simulink model "BDotv1"  (R2023b)
settings: Solver=FixedStepAuto  StartTime=0.0  StopTime=6000  FixedStep=1  RelTol=1e-3
undefined symbols (not defined in the file or in its folder): EIGEN, GL04C, IAU
libraries: aerolibtransform2 x3, aerolibutil x3, sharedutil x1, vrlib x1
settings Model: Creator=moonr  LastModifiedBy=moonr
settings HardwareCC: ProdBitPerLong=64  ProdLargestAtomicFloat=None  ProdHWDeviceType=AMD->Athlon 64

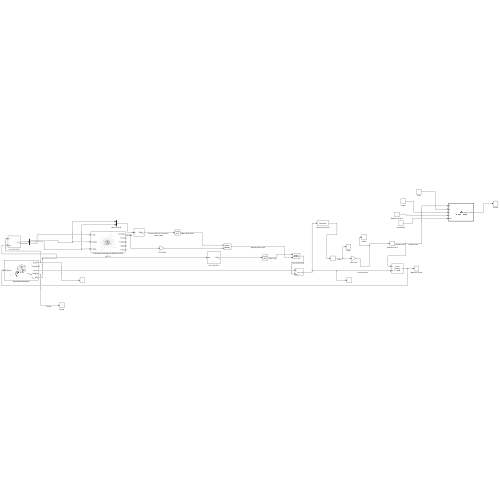
[thumbnail: Simulink's stored preview of the top-level diagram]
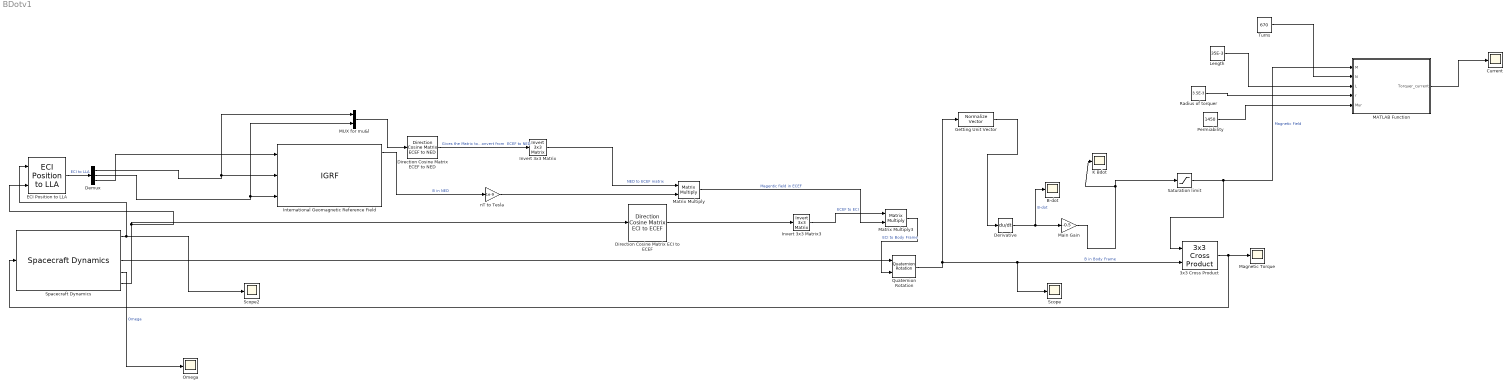
== system BDotv1 ==
  3x3 Cross Product : sharedutil/3x3 Cross Product  aMode=aMode
      settings: LibrarySourceBlock=aerolibutil/3x3 Cross Product
  B-dot : Scope
  Current : Scope
  Demux : Demux  Outputs=3
  Derivative : Derivative
  Direction Cosine Matrix ECEF to NED : aerolibtransform2/Direction Cosine Matrix ECEF to NED
  Direction Cosine Matrix ECI to ECEF : aerolibtransform2/Direction Cosine Matrix ECI to ECEF  red=IAU-2000/2006  year=2020  month=January  day=1  hour=0  min=0  sec=0  deltaT=Sec  errorflag=Error  extraparamflag=off
      settings: AttributesFormatString=%<red>
  ECI Position to LLA : aerolibtransform2/ECI Position to LLA  red=IAU-2000/2006  year=2020  month=January  day=1  hour=0  min=0  sec=0  deltaT=Day  errorflag=Error  extraparamflag=off  eunits=Metric (MKS)  earthmodel=WGS84  flat=1/298.257223563  eqradius=6378137
      settings: AttributesFormatString=%<red>
  Getting Unit Vector : vrlib/Utilities/Normalize Vector  maxzero=0
  International Geomagnetic Reference Field : IGRF  time_in=off  month=January  day=1  year=2020  sv_out=off
      settings: AttributesFormatString=%<generation>
  Invert 3x3 Matrix : aerolibutil/Invert  3x3 Matrix
  Invert 3x3 Matrix3 : aerolibutil/Invert  3x3 Matrix
  K Bdot : Scope
  Length : Constant  Value=35E-3
  MATLAB Function : MATLAB Function  TreatAsAtomicUnit=on
  MUX for mu&l : Mux  Inputs=2
  Magnetic Torque : Scope
  Main Gain : Gain  Gain=-0.5
  Matrix Multiply : Product  Multiplication=Matrix(*)
  Matrix Multiply3 : Product  Multiplication=Matrix(*)
  "Omega " : Scope
  Permiability : Constant  Value=1450
  Quaternion Rotation : aerolibutil/Quaternion Rotation
  Radius of torquer : Constant  Value=3.5E-3
  Saturation limit : Saturate  UpperLimit=[0.050, 0.050, 0.050]  LowerLimit=[-0.050, -0.050, -0.050]
  Scope : Scope
  Scope2 : Scope
  Spacecraft Dynamics : SpacecraftDynamics  forcesIn=off  outportFrame=Fixed-frame  mass=2.51755  inertia=[0.01303, 0.000076172116, -0.0002044; 0.000076172116, 0.01276, 0.0005856; -0.0002044, 0.0005856, 0.00425]  stateFormatNum=ICRF state vector  attitudeRate=[10, 10, 10]  useGravGrad=off  earthSH=EIGEN-GL04C  useEphemerisDateRange=off
  Turns : Constant  Value=670
  nT to Tesla : Gain  Gain=1e-9
  wires:
  Spacecraft Dynamics/1 -> Scope2/1, ECI Position to LLA/1
  ECI Position to LLA/1 -> Demux/1  "ECI to LLA"
  Demux/1 -> MUX for mu&l/1, International Geomagnetic Reference Field/2
  Demux/2 -> MUX for mu&l/2, International Geomagnetic Reference Field/3
  Demux/3 -> International Geomagnetic Reference Field/1
  Direction Cosine Matrix ECEF to NED/1 -> Invert 3x3 Matrix/1  "Gives the Matrix to convert from  ECEF to NED"
  Matrix Multiply/1 -> Matrix Multiply3/2  "Magentic field in ECEF"
  Spacecraft Dynamics/5 -> Direction Cosine Matrix ECI to ECEF/1, ECI Position to LLA/2
  Spacecraft Dynamics/4 -> "Omega "/1  "Omega"
  MUX for mu&l/1 -> Direction Cosine Matrix ECEF to NED/1
  Direction Cosine Matrix ECI to ECEF/1 -> Invert 3x3 Matrix3/1
  Invert 3x3 Matrix3/1 -> Matrix Multiply3/1  "ECEF to ECI"
  Quaternion Rotation/1 -> Getting Unit Vector/1, Scope/1, 3x3 Cross Product/2  "B in Body Frame"
  Derivative/1 -> B-dot/1, Main Gain/1  "B-dot"
  Main Gain/1 -> Saturation limit/1, K Bdot/1
  International Geomagnetic Reference Field/1 -> nT to Tesla/1  "B in NED"
  Invert 3x3 Matrix/1 -> Matrix Multiply/1  "NED to ECEF matrix"
  3x3 Cross Product/1 -> Spacecraft Dynamics/1, Magnetic Torque/1
  nT to Tesla/1 -> Matrix Multiply/2
  Spacecraft Dynamics/3 -> Quaternion Rotation/1
  Matrix Multiply3/1 -> Quaternion Rotation/2  "ECI to Body Frame"
  Saturation limit/1 -> 3x3 Cross Product/1, MATLAB Function/1(M)  "Magnetic Field"
  Turns/1 -> MATLAB Function/2(N)
  Length/1 -> MATLAB Function/3(L)
  Radius of torquer/1 -> MATLAB Function/4(r)
  Permiability/1 -> MATLAB Function/5(Mur)
  MATLAB Function/1(Torquer_current) -> Current/1
  Getting Unit Vector/1 -> Derivative/1

== matlab function BDotv1/MATLAB Function ==
  data: M input; Torquer_current output; N input; L input; r input; Mur input

%Date-11/2/24
%Ur(mu-r) for SS-430FR = 1450 
% We take radius=2.75mm to 3.5mm=r
% Thereby number of turns=1232-670=N
%Length of the Torquer=35mm=L
%Formula returns Current required as a function of Magnetic Dipole and
%turns

%Formula is
%Torquer_current=(M*(1+(Mur-1)*Nd))/(pi*r^2*N*(1+(Mur-1)*Nd)+(Mur-1))


function Torquer_current  = Torquer_current(M,N,L,r,Mur)

%Mur=1450;
piVal = pi;
Nd = Demag_factor(L,r);

Torquer_current = (M*(1+(Mur-1)*Nd))/( piVal*r^2*N* (((Mur-1)*Nd)+Mur));

end
